simulink model "Kinarm_Approach_Avoidance_Task"  (R2019b)
settings: Solver=ode4  StartTime=0.0  StopTime=inf  FixedStep=BKIN_STEP_TIME  RelTol=1e-3  EnableMultiTasking=on
StartFcn:
  |  warndlg('Dexterit-E models cannot run under simulation. Please compile your model and run it from within Dexterit-E.');set_param(bdroot,'SimulationCommand','stop')
model workspace (MAT data in the model file):
  ADJUST_START = 2
  APPROACH_TARGET_COL = 6
  AVOID_DIST_ADJUST = 6
  AVOID_TARGET_COL = 2
  BEGIN_TARGET_COL = 3
  BKIN_KINEMATIC_FRAME_SIZE = 400
  BKIN_STEP_TIME = 0.00025
  COLOUR_2ND = 7
  COLOUR_3RD = 11
  COLOUR_4TH = 12
  COLOUR_INIT = 6
  CS_OR_AS = 7
  ERROR_DELAY = 10
  E_ACTIVE_APP = 24
  E_APPROACHED = 19
  E_AVOIDED = 21
  E_CIRCLE_APP = 26
  E_ERROR_TRIAL = 23
  E_HAND_IN_START = 17
  E_HAND_LEFT = 16
  E_LEFT_TARG_ON = 2
  E_LOC_1 = 3
  E_LOC_10 = 12
  E_LOC_11 = 13
  E_LOC_12 = 14
  E_LOC_2 = 4
  E_LOC_3 = 5
  E_LOC_4 = 6
  E_LOC_5 = 7
  E_LOC_6 = 8
  E_LOC_7 = 9
  E_LOC_8 = 10
  E_LOC_9 = 11
  E_NO_EVENT = 0
  E_RIGHT_TARG_ON = 1
  E_SEDEN_APP = 25
  E_SQUARE_APP = 27
  E_TARGET_ON = 18
  E_TIMED_OUT = 22
  E_TRIAL_END = 20
  E_TRIAL_START = 15
  INFO_TARGET_COL = 5
  LABEL_COL = 4
  LABEL_HEIGHT = 9
  LABEL_TEXT = 8
  LENGTH = 3
  MAX_FORCE = 3
  MAX_FORCE_BG = 4
  RADIUS_VIS = 3
  RAMP_DURATION = 5
  RAND_START_DELAY = 8
  REACH_TIME = 11
  START_HOLD_DELAY = 7
  START_TARGET_COL = 1
  STROKE_WIDTH = 10
  SUCCESS_DELAY = 9
  TARGET_X = 4
  TARGET_Y = 5
  TARG_DIST = 1
  TARG_LENGTH = 3
  TARG_WIDTH = 4
  TOGGLE_FIELD = 8
  TRIAL_TIME = 12
  WIDTH = 4
  Width = 4
  col_x = 1
  col_y = 2
undefined symbols (not defined in the file): slselsubs
libraries: Video x7, General x3, KINARM_general x3, KINARM_EP_loads x3
settings Model: ModifiedComment=chris -- Wed Feb 16 09:18:30 2005 -- Version 1.1384  ModifiedHistory=Feb 16/05 - Add error repeat, add offset ramp  ExtModeArmWhenConnect=off  ExtModeLogAll=off  OrderedModelArguments=off  Creator=Chris Grebeldinger  LastModifiedBy=User
settings SolverCC: AutoInsertRateTranBlk=on
settings DataIOCC: SaveFormat=Array  SignalLoggingSaveFormat=ModelDataLogs  SaveOutput=off  SaveTime=off  ReturnWorkspaceOutputs=off  SignalLoggingName=sigsOut
settings OptimizationCC: BlockReduction=off  BooleanDataType=off  OptimizeBlockIOStorage=off  BufferReuse=off  GlobalBufferReuse=off  ExpressionFolding=off  ExpressionDepthLimit=2147483647  LocalBlockOutputs=off  InitFltsAndDblsToZero=on  LifeSpan=inf  OptimizeDataStoreBuffers=off  BusAssignmentInplaceUpdate=off
settings DebuggingCC: SaveWithParameterizedLinksMsg=none  UnderspecifiedInitializationDetection=Classic  MergeDetectMultiDrivingBlocksExec=none  SignalResolutionControl=TryResolveAllWithWarning  MultiTaskDSMMsg=warning  FcnCallInpInsideContextMsg=warning  BusObjectLabelMismatch=none  StateNameClashWarn=warning  StrictBusMsg=ErrorOnBusTreatedAsVector  SFUnexpectedBacktrackingDiag=warning  SFNoUnconditionalDefaultTransitionDiag=warning  SFExecutionAtInitializationDiag=none  ArithmeticOperatorsInVariantConditions=warning
settings HardwareCC: ProdBitPerPointer=32  ProdBitPerSizeT=32  ProdBitPerPtrDiffT=32  ProdLargestAtomicFloat=None  ProdWordSize=32  ProdLongLongMode=on  ProdHWDeviceType=Generic->32-bit x86 compatible  TargetLongLongMode=on  TargetIntDivRoundTo=Zero  TargetEndianess=LittleEndian  TargetHWDeviceType=Generic->32-bit x86 compatible
settings ModelReferenceCC: PropagateSignalLabelsOutOfModel=off
settings SFSimCC: SimCustomHeaderCode="#include \"stdlib.h\""  SimUseLocalCustomCode=off  SimParseCustomCode=off  CustomCodeUndefinedFunction=UseInterfaceOnly
settings RTWCC: Description=Simulink Real-Time  SystemTargetFile=slrt.tlc  TemplateMakefile=slrt_default_tmf  RTWUseLocalCustomCode=off  CustomSourceCode="#include \"stdlib.h\""  CodeExecutionProfiling=on
settings CodeAppCC: MaxIdLength=63  StateflowObjectComments=on
settings SimulinkRealTimeCC: TargetFcnLib=ansi_tfl_tmw.mat  GeneratePreprocessorConditionals=Disable all  PreserveStateflowLocalDataDimensions=off
settings ConfigComp: CovMetricSettings=dw  CovHtmlReporting=on  CovSaveCumulativeToWorkspaceVar=on  CovSaveSingleToWorkspaceVar=on  CovExternalEMLEnable=off

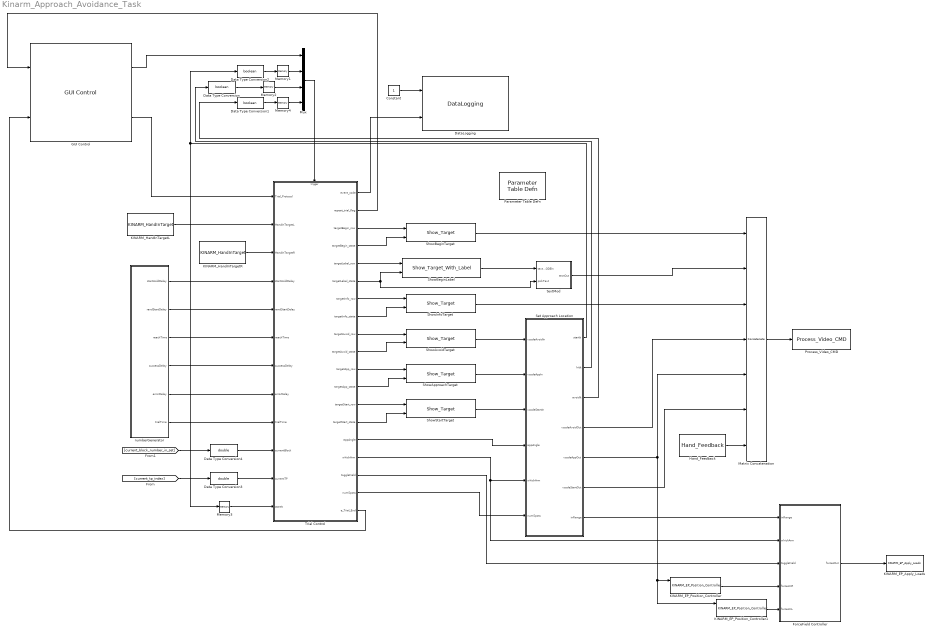
== system Kinarm_Approach_Avoidance_Task ==
  Constant : Constant
  Data Type Conversion : DataTypeConversion  OutDataTypeStr=boolean
  Data Type Conversion1 : DataTypeConversion  OutDataTypeStr=boolean
  Data Type Conversion2 : DataTypeConversion  OutDataTypeStr=boolean
  Data Type Conversion3 : DataTypeConversion  OutDataTypeStr=double
  Data Type Conversion4 : DataTypeConversion  OutDataTypeStr=double
  DataLogging : General/DataLogging  log_event_codes=on  log_analog_inputs=off  show_time_remaining=off  ecat_include=on
  ForceField Controller : Subsystem
  GUI Control : General/GUI Control  task_version=1.0  show_repeat_trial_flag=on  use_custom_tp=off  target_type_str=Circle  Target_Type=1  XYcols=[1 2]  Vcols=3  Lcols=4  indices_padding=[0 0 0 0;0 0 0 0]  target_table_rows=64  load_table_rows=20  tp_table_rows=100
  Hand_Feedback : KINARM_general/Hand_Feedback  feedback_cntl_src=none
  KINARM_EP_Apply_Loads : KINARM_EP_loads/KINARM_EP_Apply_Loads  up_duration=1500  down_duration=1500  max_force=30
  KINARM_EP_Position_Controller : KINARM_EP_loads/KINARM_EP_Position_Controller  use_dom_hand=on  inertias_for_FF=KINARM End Point robot  gain_choice=Standard Movement  sample_time=0.001
  KINARM_EP_Position_Controller1 : KINARM_EP_loads/KINARM_EP_Position_Controller  use_dom_hand=off  inertias_for_FF=KINARM End Point robot  gain_choice=Standard Movement  sample_time=0.001
  KINARM_HandInTargetL : KINARM_general/KINARM_HandInTarget  use_dominant_hand=off  target_type=Circle  num_states=1  attribcol1=[RADIUS_VIS]  attribcol2=[0]  attribcol3=[0]  attribcol4=[0]  attribcol5=[0]
  KINARM_HandInTargetR : KINARM_general/KINARM_HandInTarget  use_dominant_hand=on  target_type=Circle  num_states=1  attribcol1=[RADIUS_VIS]  attribcol2=[0]  attribcol3=[0]  attribcol4=[0]  attribcol5=[0]
  Matrix Concatenation : Concatenate  NumInputs=7  Mode=Multidimensional array
  Memory{1..4} (4 alike) : Memory
  Mux : Mux
  Parameter Table Defn : General/Parameter Table Defn  ShowInLibBrowser=0
  Process_Video_CMD : Video/Process_Video_CMD  video_delay=50
  Set Approach Location : Subsystem
  ShowApproachTarget : Video/Show_Target  target_type=Circle  num_states=1  attribcol1=[COLOUR_INIT 0 0 RADIUS_VIS]  attribcol2=[0 0 0 0]  attribcol3=[0 0 0 0]  attribcol4=[0 0 0 0]  attribcol5=[0 0 0 0]  stateindices_padding=[0 0 0 0 0 0 0;0 0 0 0 0 0 0;0 0 0 0 0 0 0;0 0 0 0 0 0 0;0 0 0 0 0 0 0]  source=dialog  opacity=100  target_display=Both subject and operator displays  num_col=4
  ShowAvoidTarget : Video/Show_Target  target_type=Circle  num_states=1  attribcol1=[COLOUR_INIT COLOUR_2ND STROKE_WIDTH RADIUS_VIS]  attribcol2=[0 0 0 0]  attribcol3=[0 0 0 0]  attribcol4=[0 0 0 0]  attribcol5=[0 0 0 0]  stateindices_padding=[0 0 0 0 0 0 0;0 0 0 0 0 0 0;0 0 0 0 0 0 0;0 0 0 0 0 0 0;0 0 0 0 0 0 0]  source=dialog  opacity=100  target_display=Both subject and operator displays  num_col=4
  ShowBeginLabel : Video/Show_Target_With_Label  target_type=Circle  num_states=3  attribcol1=[0 0 0 0 LABEL_TEXT COLOUR_INIT LABEL_HEIGHT]  attribcol2=[0 0 0 0 LABEL_TEXT COLOUR_2ND LABEL_HEIGHT]  attribcol3=[0 0 0 0 LABEL_TEXT COLOUR_3RD LABEL_HEIGHT]  attribcol4=[0 0 0 0 0 0 0]  attribcol5=[0 0 0 0 0 0 0]  stateindices_padding=[0 0 0 0;0 0 0 0;0 0 0 0;0 0 0 0;0 0 0 0]  source=dialog  opacity=100  target_display=Both subject and operator displays
  ShowBeginTarget : Video/Show_Target  target_type=Circle  num_states=1  attribcol1=[COLOUR_INIT COLOUR_2ND STROKE_WIDTH RADIUS_VIS]  attribcol2=[0 0 0 0]  attribcol3=[0 0 0 0]  attribcol4=[0 0 0 0]  attribcol5=[0 0 0 0]  stateindices_padding=[0 0 0 0 0 0 0;0 0 0 0 0 0 0;0 0 0 0 0 0 0;0 0 0 0 0 0 0;0 0 0 0 0 0 0]  source=dialog  opacity=100  target_display=Both subject and operator displays  num_col=4
  ShowInfoTarget : Video/Show_Target  target_type=Rectangle  num_states=4  attribcol1=[COLOUR_INIT 0 0 TARGET_X TARGET_Y 0]  attribcol2=[COLOUR_2ND 0 0 TARGET_X TARGET_Y 0]  attribcol3=[COLOUR_3RD 0 0 TARGET_X TARGET_Y 0]  attribcol4=[COLOUR_4TH 0 0 TARGET_X TARGET_Y 0]  attribcol5=[0 0 0 0 0 0]  stateindices_padding=[0 0 0 0 0;0 0 0 0 0;0 0 0 0 0;0 0 0 0 0;0 0 0 0 0]  source=dialog  opacity=100  target_display=Both subject and operator displays  num_col=6
  ShowStartTarget : Video/Show_Target  target_type=Circle  num_states=1  attribcol1=[COLOUR_INIT 0 0 RADIUS_VIS]  attribcol2=[0 0 0 0]  attribcol3=[0 0 0 0]  attribcol4=[0 0 0 0]  attribcol5=[0 0 0 0]  stateindices_padding=[0 0 0 0 0 0 0;0 0 0 0 0 0 0;0 0 0 0 0 0 0;0 0 0 0 0 0 0;0 0 0 0 0 0 0]  source=dialog  opacity=100  target_display=Both subject and operator displays  num_col=4
  Trial Control : Stateflow chart  TreatAsAtomicUnit=on
  numberGenerator : Subsystem
  textMod : Subsystem
  wires:
  Trial Control/19(e_Trial_End) -> GUI Control/2
  Trial Control/14(targetStart_state) -> ShowStartTarget/2
  Trial Control/13(targetStart_row) -> ShowStartTarget/1
  Matrix Concatenation/1 -> Process_Video_CMD/1
  Trial Control/1(event_code) -> DataLogging/2
  ShowStartTarget/1 -> Set Approach Location/3(vcodeStartIn)
  Constant/1 -> DataLogging/1
  GUI Control/2 -> Trial Control/1(Trial_Protocol)
  Trial Control/11(targetApp_row) -> ShowApproachTarget/1
  Trial Control/12(targetApp_state) -> ShowApproachTarget/2
  Trial Control/2(repeat_trial_flag) -> GUI Control/1
  KINARM_EP_Position_Controller/1 -> ForceField Controller/4(forcesInR)
  GUI Control/1 -> Mux/1
  [current_tp_index] -> Data Type Conversion3/1
  ShowApproachTarget/1 -> Set Approach Location/2(vcodeAppIn)
  Set Approach Location/6(vcodeStartOut) -> Matrix Concatenation/6
  Set Approach Location/5(vcodeAppOut) -> KINARM_EP_Position_Controller/1, KINARM_EP_Position_Controller1/1, Matrix Concatenation/5
  Set Approach Location/4(vcodeAvoidOut) -> Matrix Concatenation/4
  Set Approach Location/1(startIt) -> Memory3/1, Data Type Conversion2/1
  KINARM_EP_Position_Controller1/1 -> ForceField Controller/5(forcesInL)
  Trial Control/15(appAngle) -> Set Approach Location/4(appAngle)
  Trial Control/16(whichArm) -> ForceField Controller/2(whichArm), Set Approach Location/5(whichArm)
  ShowInfoTarget/1 -> Matrix Concatenation/3
  KINARM_HandInTargetR/1 -> Trial Control/3(HandInTargetR)
  KINARM_HandInTargetL/1 -> Trial Control/2(HandInTargetL)
  Trial Control/17(toggleField) -> ForceField Controller/3(toggleField)
  ForceField Controller/1(forcesOut) -> KINARM_EP_Apply_Loads/1
  Trial Control/3(targetBegin_row) -> ShowBeginTarget/1
  Trial Control/4(targetBegin_state) -> ShowBeginTarget/2
  Trial Control/7(targetInfo_row) -> ShowInfoTarget/1
  Trial Control/8(targetInfo_state) -> ShowInfoTarget/2
  Trial Control/5(targetLabel_row) -> ShowBeginLabel/1
  Trial Control/6(targetLabel_state) -> ShowBeginLabel/2, textMod/2(pickText)
  numberGenerator/1(startHoldDelay) -> Trial Control/4(startHoldDelay)
  numberGenerator/2(randStartDelay) -> Trial Control/5(randStartDelay)
  numberGenerator/6(trialTime) -> Trial Control/9(trialTime)
  numberGenerator/3(reachTime) -> Trial Control/6(reachTime)
  numberGenerator/4(successDelay) -> Trial Control/7(successDelay)
  numberGenerator/5(errorDelay) -> Trial Control/8(errorDelay)
  ShowBeginLabel/1 -> textMod/1(textVCODEIn)
  ShowBeginTarget/1 -> Matrix Concatenation/1
  Hand_Feedback/1 -> Matrix Concatenation/7
  Set Approach Location/7(inRange) -> ForceField Controller/1(inRange)
  Mux/1 -> Trial Control/Trigger
  Memory2/1 -> Mux/3
  Memory4/1 -> Mux/4
  Set Approach Location/2(hitIt) -> Data Type Conversion/1
  Set Approach Location/3(avoidIt) -> Data Type Conversion1/1
  Data Type Conversion/1 -> Memory2/1
  Data Type Conversion1/1 -> Memory4/1
  Data Type Conversion2/1 -> Memory1/1
  Memory1/1 -> Mux/2
  Data Type Conversion3/1 -> Trial Control/11(currentTP)
  Trial Control/9(targetAvoid_row) -> ShowAvoidTarget/1
  Trial Control/10(targetAvoid_state) -> ShowAvoidTarget/2
  ShowAvoidTarget/1 -> Set Approach Location/1(vcodeAvoidIn)
  [current_block_number_in_set] -> Data Type Conversion4/1
  Data Type Conversion4/1 -> Trial Control/10(currentBlock)
  Memory3/1 -> Trial Control/12(startIt)
  textMod/1(textOut) -> Matrix Concatenation/2
  Trial Control/18(numSpots) -> Set Approach Location/6(numSpots)

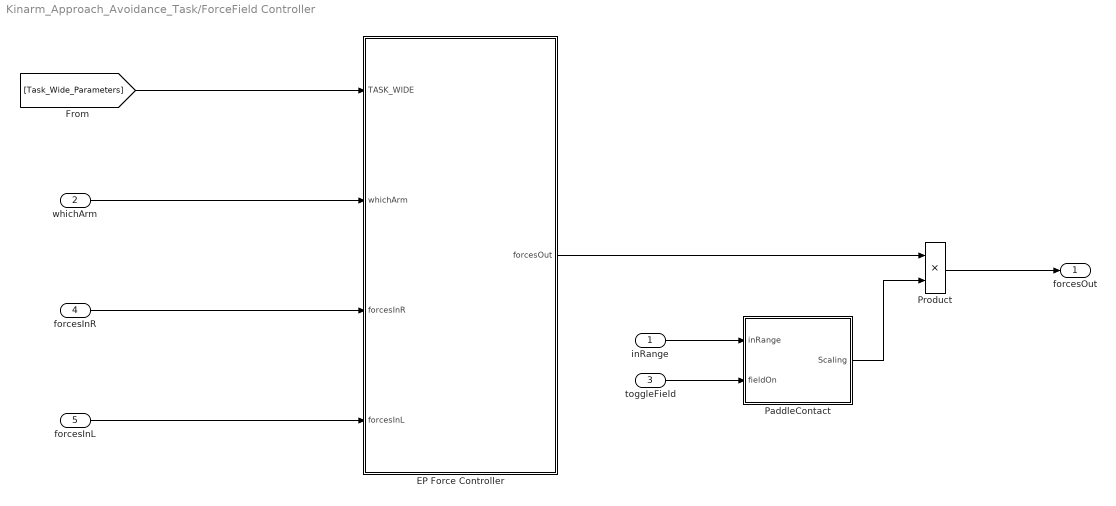
== system Kinarm_Approach_Avoidance_Task/ForceField Controller ==
  inRange : Inport
  whichArm : Inport  Port=2
  toggleField : Inport  Port=3
  forcesInR : Inport  Port=4
  forcesInL : Inport  Port=5
  EP Force Controller : MATLAB Function  TreatAsAtomicUnit=on
  PaddleContact : Subsystem  mask(Perturbation){}
  Product : Product
  forcesOut : Outport
  wires:
  [Task_Wide_Parameters] -> EP Force Controller/1(TASK_WIDE)
  EP Force Controller/1(forcesOut) -> Product/1
  toggleField/1 -> PaddleContact/2(fieldOn)
  forcesInR/1 -> EP Force Controller/3(forcesInR)
  whichArm/1 -> EP Force Controller/2(whichArm)
  forcesInL/1 -> EP Force Controller/4(forcesInL)
  PaddleContact/1(Scaling) -> Product/2
  inRange/1 -> PaddleContact/1(inRange)
  Product/1 -> forcesOut/1

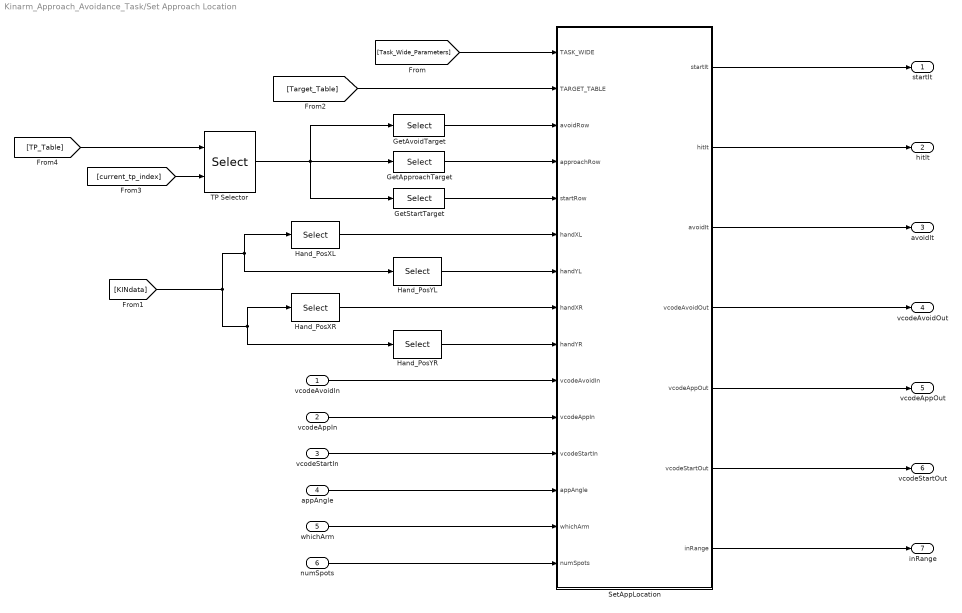
== system Kinarm_Approach_Avoidance_Task/Set Approach Location ==
  vcodeAvoidIn : Inport
  vcodeAppIn : Inport  Port=2
  vcodeStartIn : Inport  Port=3
  appAngle : Inport  Port=4
  whichArm : Inport  Port=5
  numSpots : Inport  Port=6
  GetApproachTarget : Selector  NumberOfDimensions=2  InputPortWidth=3  IndexOptions=Select all,Index vector (dialog)  Indices=[1],[APPROACH_TARGET_COL]  OutputSizes=slselsubs([(-2),(-2)],1),slselsubs([(-2),(-2)],2)
  GetAvoidTarget : Selector  NumberOfDimensions=2  InputPortWidth=3  IndexOptions=Select all,Index vector (dialog)  Indices=[1],[AVOID_TARGET_COL]  OutputSizes=slselsubs([(-2),(-2)],1),slselsubs([(-2),(-2)],2)
  GetStartTarget : Selector  NumberOfDimensions=2  InputPortWidth=3  IndexOptions=Select all,Index vector (dialog)  Indices=[1],[START_TARGET_COL]  OutputSizes=slselsubs([(-2),(-2)],1),slselsubs([(-2),(-2)],2)
  Hand_PosXL : Selector  NumberOfDimensions=2  InputPortWidth=3  IndexOptions=Index vector (dialog),Index vector (dialog)  Indices=[2],[23]  OutputSizes=slselsubs([(-2),(-2)],1),slselsubs([(-2),(-2)],2)
  Hand_PosXR : Selector  NumberOfDimensions=2  InputPortWidth=3  IndexOptions=Index vector (dialog),Index vector (dialog)  Indices=[1],[23]  OutputSizes=slselsubs([(-2),(-2)],1),slselsubs([(-2),(-2)],2)
  Hand_PosYL : Selector  NumberOfDimensions=2  InputPortWidth=3  IndexOptions=Index vector (dialog),Index vector (dialog)  Indices=[2],[24]  OutputSizes=slselsubs([(-2),(-2)],1),slselsubs([(-2),(-2)],2)
  Hand_PosYR : Selector  NumberOfDimensions=2  InputPortWidth=3  IndexOptions=Index vector (dialog),Index vector (dialog)  Indices=[1],[24]  OutputSizes=slselsubs([(-2),(-2)],1),slselsubs([(-2),(-2)],2)
  SetAppLocation : MATLAB Function  TreatAsAtomicUnit=on
  TP Selector : Selector  NumberOfDimensions=2  InputPortWidth=3  IndexOptions=Index vector (port),Select all  Indices=1,-1  OutputSizes=slselsubs([(-2),(-2)],1),slselsubs([(-2),(-2)],2)
  startIt : Outport
  hitIt : Outport  Port=2
  avoidIt : Outport  Port=3
  vcodeAvoidOut : Outport  Port=4
  vcodeAppOut : Outport  Port=5
  vcodeStartOut : Outport  Port=6
  inRange : Outport  Port=7
  wires:
  [Task_Wide_Parameters] -> SetAppLocation/1(TASK_WIDE)
  [current_tp_index] -> TP Selector/2
  Hand_PosXL/1 -> SetAppLocation/6(handXL)
  Hand_PosYL/1 -> SetAppLocation/7(handYL)
  [TP_Table] -> TP Selector/1
  TP Selector/1 -> GetStartTarget/1, GetApproachTarget/1, GetAvoidTarget/1
  GetApproachTarget/1 -> SetAppLocation/4(approachRow)
  [Target_Table] -> SetAppLocation/2(TARGET_TABLE)
  SetAppLocation/2(hitIt) -> hitIt/1
  vcodeAvoidIn/1 -> SetAppLocation/10(vcodeAvoidIn)
  SetAppLocation/4(vcodeAvoidOut) -> vcodeAvoidOut/1
  vcodeAppIn/1 -> SetAppLocation/11(vcodeAppIn)
  vcodeStartIn/1 -> SetAppLocation/12(vcodeStartIn)
  SetAppLocation/5(vcodeAppOut) -> vcodeAppOut/1
  SetAppLocation/6(vcodeStartOut) -> vcodeStartOut/1
  GetAvoidTarget/1 -> SetAppLocation/3(avoidRow)
  GetStartTarget/1 -> SetAppLocation/5(startRow)
  Hand_PosXR/1 -> SetAppLocation/8(handXR)
  Hand_PosYR/1 -> SetAppLocation/9(handYR)
  [KINdata] -> Hand_PosYL/1, Hand_PosXL/1, Hand_PosYR/1, Hand_PosXR/1
  SetAppLocation/1(startIt) -> startIt/1
  SetAppLocation/3(avoidIt) -> avoidIt/1
  whichArm/1 -> SetAppLocation/14(whichArm)
  appAngle/1 -> SetAppLocation/13(appAngle)
  numSpots/1 -> SetAppLocation/15(numSpots)
  SetAppLocation/7(inRange) -> inRange/1

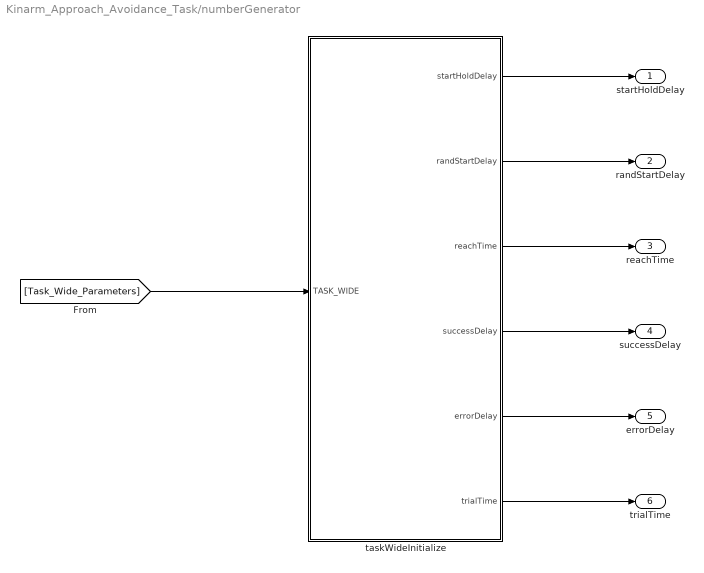
== system Kinarm_Approach_Avoidance_Task/numberGenerator ==
  taskWideInitialize : MATLAB Function  TreatAsAtomicUnit=on
  startHoldDelay : Outport
  randStartDelay : Outport  Port=2
  reachTime : Outport  Port=3
  successDelay : Outport  Port=4
  errorDelay : Outport  Port=5
  trialTime : Outport  Port=6
  wires:
  [Task_Wide_Parameters] -> taskWideInitialize/1(TASK_WIDE)
  taskWideInitialize/1(startHoldDelay) -> startHoldDelay/1
  taskWideInitialize/2(randStartDelay) -> randStartDelay/1
  taskWideInitialize/6(trialTime) -> trialTime/1
  taskWideInitialize/3(reachTime) -> reachTime/1
  taskWideInitialize/4(successDelay) -> successDelay/1
  taskWideInitialize/5(errorDelay) -> errorDelay/1

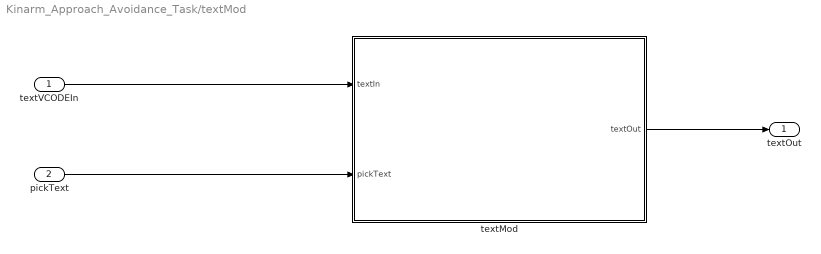
== system Kinarm_Approach_Avoidance_Task/textMod ==
  textVCODEIn : Inport
  pickText : Inport  Port=2
  textMod : MATLAB Function  TreatAsAtomicUnit=on
  textOut : Outport
  wires:
  textMod/1(textOut) -> textOut/1
  textVCODEIn/1 -> textMod/1(textIn)
  pickText/1 -> textMod/2(pickText)

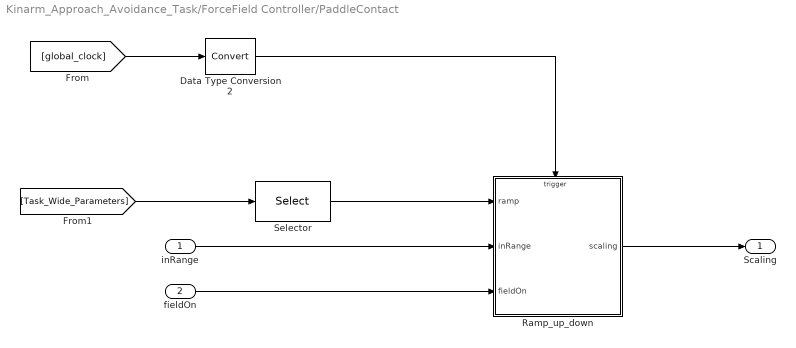
== system Kinarm_Approach_Avoidance_Task/ForceField Controller/PaddleContact ==
  inRange : Inport
  fieldOn : Inport  Port=2
  Data Type Conversion2 : DataTypeConversion
  Ramp_up_down : Stateflow chart  TreatAsAtomicUnit=on
  Selector : Selector  NumberOfDimensions=2  InputPortWidth=3  IndexOptions=Index vector (dialog),Select all  Indices=[RAMP_DURATION],[3]  OutputSizes=slselsubs([(-2),(-2)],1),1
  Scaling : Outport
  wires:
  Ramp_up_down/1(scaling) -> Scaling/1
  [global_clock] -> Data Type Conversion2/1
  Data Type Conversion2/1 -> Ramp_up_down/Trigger
  [Task_Wide_Parameters] -> Selector/1
  Selector/1 -> Ramp_up_down/1(ramp)
  inRange/1 -> Ramp_up_down/2(inRange)
  fieldOn/1 -> Ramp_up_down/3(fieldOn)

== matlab function Kinarm_Approach_Avoidance_Task/Set Approach Location/SetAppLocation ==
  data: startIt output; hitIt output; avoidIt output; vcodeAvoidOut output; vcodeAppOut output; vcodeStartOut output; TASK_WIDE input; TARGET_TABLE input; avoidRow input; approachRow input; startRow input; handXL input; handYL input; handXR input; handYR input; vcodeAvoidIn input; vcodeAppIn input; vcodeStartIn input; appAngle input; whichArm input; numSpots input; TARG_DIST parameter; RADIUS_VIS parameter; ADJUST_START parameter; inRange output
function [startIt, hitIt, avoidIt, vcodeAvoidOut, vcodeAppOut, vcodeStartOut, inRange] = fcn...
    (TASK_WIDE, TARGET_TABLE, avoidRow, approachRow, startRow, handXL, handYL, handXR, handYR, vcodeAvoidIn, vcodeAppIn, vcodeStartIn, appAngle, whichArm, numSpots,...
    TARG_DIST, RADIUS_VIS, ADJUST_START)
%This function checks if the hand is in start, approach, or avoid targets.

%% initialize hand and location to be displayed
targDist = TASK_WIDE(TARG_DIST); %gets distance of targets set from task wide
adjustStart = TASK_WIDE(ADJUST_START); %adjusts the left and right distance from the midline for the center of start/approach/avoid targets
angleArray = [0:2*pi/numSpots:2*pi-2*pi/numSpots]; %get radians for each location

%assume hand is right hand being tested
handX = handXR;
handY = handYR;
whichLoc = angleArray(appAngle); %get the location

if (whichArm == 1) %1 is left arm, left arm is being tested
	adjustStart = -TASK_WIDE(ADJUST_START); %shift target center to the left
    handX = handXL;
    handY = handYL;
end

%% initialize radius

rValStart = TARGET_TABLE(startRow,RADIUS_VIS)*0.01; %radius of start target
rValApp = TARGET_TABLE(approachRow,RADIUS_VIS)*0.01; %radius of approach target
rValApp2 = targDist*0.01-rValStart; %radius of force field around approach target accounts for starting target
rValAvoid = TARGET_TABLE(avoidRow,RADIUS_VIS)*0.01; %radius of avoid target

%% change vcodes for start target contact
%Checks if hand is inside of start target (circle) and shamelessly stolen 
%from HandInTarget block and simplified.
vcodeStartOut = vcodeStartIn;

vcodeStartOut(3) = vcodeStartIn(3) + adjustStart*0.01; %x position adjusted depending on arm assessed
vcodeStartOut(4) = vcodeStartIn(4);

deltaxStart=handX-vcodeStartOut(3); %find difference between hand and approach target
deltayStart=handY-vcodeStartOut(4);

distanceStart = deltaxStart.^2 + deltayStart.^2;

if (distanceStart <= rValStart^2) %if hand is in start target then trigger start
    startIt = 1;
else
    startIt = 0;
end


%% change vcodes for approach target contact
%Same as above but for approach target (circle).
vcodeAppOut = vcodeAppIn;

vcodeAppOut(3) = vcodeAppIn(3) + targDist*cos(whichLoc)*0.01 + adjustStart*0.01;
vcodeAppOut(4) = vcodeAppIn(4) + targDist*sin(whichLoc)*0.01;

deltaxApp=handX-vcodeAppOut(3);
deltayApp=handY-vcodeAppOut(4);

distanceApp = deltaxApp.^2 + deltayApp.^2;
if (distanceApp < rValApp^2) %if hand inside approach target
    hitIt = 1;
else
    hitIt = 0;
end

if (distanceApp < rValApp2^2) %if hand inside approach target force field
    inRange = 1;
else
    inRange = 0;
end

%% change vcodes for avoid target no contact
%similar to above but checks if hand is inside avoid target (circle)

vcodeAvoidOut = vcodeAvoidIn;

vcodeAvoidOut(3) = vcodeAvoidIn(3) + targDist*cos(whichLoc+pi)*0.01 + adjustStart*0.01;
vcodeAvoidOut(4) = vcodeAvoidIn(4) + targDist*sin(whichLoc+pi)*0.01;

deltaxAvoid=handX-vcodeAvoidOut(3);
deltayAvoid=handY-vcodeAvoidOut(4);

distanceAvoid = deltaxAvoid.^2 + deltayAvoid.^2;
if (distanceAvoid < rValAvoid^2) %if hand inside approach target
    avoidIt = 1;
else
    avoidIt = 0;
end

== stateflow chart Kinarm_Approach_Avoidance_Task/Trial Control ==
  state Initialize/
    %Task checks if the participant reached for a certain trial or avoided
    %a certain trial successfully,
    %blocks must be 48 trials long
    %each block must have the same type of TP (1-12 or 13-24)
    entry:
    targetStart_row = Trial_Protocol(START_TARGET_COL);
    targetStart_state = 0; %target for beginning a trial
    targetApp_state = 0; %approach target
    targetAvoid_state = 0; %avoid target
    targetInfo_row = Trial_Protocol(INFO_TARGET_COL); %image of approach/avoid association
    targetBegin_row = Trial_Protocol(BEGIN_TARGET_COL); %target for beginning a block
    targetLabel_row = Trial_Protocol(LABEL_COL); %target for displaying text
    targetInfo_state = 0;
  state MainTrial
    state outputBlockOrder/
      %pick 0 or 1 based on the TP to approach or avoid CS or AS images
      entry:
      appAvoidCS = mod(currentTP,2);
      appAvoidAS = mod(currentTP,2);
      csCount = 0;
      asCount = 0;
    state StartofTrial/
      %start trial
      entry:
      targetApp_row = Trial_Protocol(APPROACH_TARGET_COL);
      targetAvoid_row = Trial_Protocol(AVOID_TARGET_COL);
      holdStartTime = startHoldDelay + rand()*randStartDelay; %starting delay
      targetStart_state = 1;
      targetApp_state = 0;
      targetAvoid_state = 0;
      toggleField = 0;
      repeat_trial_flag = 0;
      targetBegin_state = 0;
      targetLabel_state = 0;
      targetInfo_state = 0;
      tpCount(currentTP) = tpCount(currentTP) + 1; %increment the tpCount
      [appAngle, whichArm, numSpots] = arraySetup(tpCount,currentTP); %call the random array of values
      event_code = 1 + whichArm; %send out event code to identify arm
    state csCount/
      entry:
      %sets the circle square condition
      csCount = csCount + 1;
      appAvoid = appAvoidCS;
      %event codes 26 and 27 output circle square instruction images
      event_code = 26+appAvoid;
      %info states 3 and 4 show circle square instruction images
      targetInfo_state = 3+appAvoid;
    state blockStart/
      %show block start targets and note block
      entry:
      blockCheck = currentBlock;
      targetBegin_state = 1;
      targetLabel_state = 1;
      tpCount = zeros(1,24);
    state left/
      %event code for hand leaving start
      entry:
      event_code = E_HAND_LEFT;
    state asCount/
      entry:
      %sets the active sedentary condition
      asCount = asCount + 1;
      appAvoid = appAvoidAS;
      %eventcode 24 and 25 output active seden instruction images
      event_code = 24+appAvoid;
      %info states 1 and 2 show active avoid instruction images
      targetInfo_state = 1+appAvoid;
    state whichSide/
      entry:
      event_code = E_HAND_IN_START;
    state Approached/
      %hand is in approach
      entry:
      event_code = E_APPROACHED;
      toggleField = 0;
    state AppOn/
      %turn on targets for reaching
      entry:
      event_code = 2 + appAngle; %send out event for location
      toggleField = Trial_Protocol(TOGGLE_FIELD); %check if trial has forcefield
      targetStart_state = 0;
      targetApp_state = 1;
      targetAvoid_state = 1;
    state Avoided/
      %hand left avoid target
      entry:
      event_code = E_AVOIDED;
      toggleField = 0;
    state checkError/
      %send out an error for being bad
      entry:
      event_code = E_ERROR_TRIAL;
      targetLabel_state = 2;
    state TimedOut/
      %too slow to reach start/app/avoid
      entry:
      event_code = E_TIMED_OUT;
      targetLabel_state = 3;
      toggleField = 0;
    state EndOfTrial/
      % Turn off targets,
      entry:
      targetStart_state = 0;
      targetAvoid_state = 0;
      targetApp_state = 0;
      toggleField = 0;
    (junction 357) -> outputBlockOrder [order 2] : %if second CS block finished
        | [csCount == 2]
    (junction 355) -> outputBlockOrder [order 2] : %if second AS block finished
        | [asCount == 2]
    outputBlockOrder -> blockStart
    blockStart -> csCount [order 2] : %if circle or square block
        | [Trial_Protocol(CS_OR_AS) == 0]
    (junction 377) -> StartofTrial [order 2] : %if left hand is in begin target
        | [HandInTargetL(targetBegin_row) == 1]
    csCount -> (junction 377)
    (junction 357) -> blockStart [order 1] : %if no CS block finished
        | [csCount == 0]
    (junction 377) -> StartofTrial [order 1] : %if right hand is in begin target
        | [HandInTargetR(targetBegin_row) == 1]
    StartofTrial -> (junction 394)
    (junction 357) -> blockStart [order 3] : %if first CS block finished
        | [csCount == 1]
        | %swap the approach avoid condition
        | {appAvoidCS = 1-appAvoidCS;}
    (junction 355) -> blockStart [order 1] : %if no AS block finished
        | [asCount == 0]
    (junction 355) -> blockStart [order 3] : %if first AS block finished
        | [asCount == 1]
        | %swap the approach avoid condition
        | {appAvoidAS = 1-appAvoidAS;}
    blockStart -> asCount [order 1] : %if active or sedentary block
        | [Trial_Protocol(CS_OR_AS) == 1]
    asCount -> (junction 377)
    left -> (junction 394)
    (junction 394) -> TimedOut [order 1] : %delay for getting to start
        | after(trialTime, msec)
    (junction 394) -> whichSide [order 2] : %checks if hand is
        | %in start
        | [startIt == 1]
    (junction 323) -> (junction 357) [order 2] : %if circle or square block
        | [Trial_Protocol(CS_OR_AS) == 0]
    whichSide -> left [order 1] : %check if hand
        | %left start
        | [startIt == 0]
    (junction 323) -> (junction 355) [order 1] : %if active or sedentary block
        | [Trial_Protocol(CS_OR_AS) == 1]
    whichSide -> AppOn [order 2] : %hand in start delay
        | after(holdStartTime,msec)
    Approached -> checkError [order 1] : %approach to negative stimulus was incorrect during avoid block
        | [(Trial_Protocol(TOGGLE_FIELD) == 1) && appAvoid == 1]
    AppOn -> Approached [order 1] : %check if hit
        | e_hit
    Approached -> checkError [order 3] : %approach to positive stimulus was incorrect during approach block
        | [(Trial_Protocol(TOGGLE_FIELD) == 0) && appAvoid == 0]
    Approached -> EndOfTrial [order 2] : %delay after successful trial
        | after(successDelay,msec)
    AppOn -> Avoided [order 2] : %check if avoided
        | e_avoid
    AppOn -> TimedOut [order 3] : %delay for reaching to target
        | after(reachTime, msec)
    Avoided -> checkError [order 1] : %avoid to negative stimulus was incorrect during approach block
        | [(Trial_Protocol(TOGGLE_FIELD) == 1) && appAvoid == 0]
    Avoided -> checkError [order 3] : %avoid to positive stimulus was incorrect during avoid block
        | [(Trial_Protocol(TOGGLE_FIELD) == 0) && appAvoid == 1]
    Avoided -> EndOfTrial [order 2] : %delay after successful trial
        | after(successDelay,msec)
    checkError -> EndOfTrial : %delay after error trial
        | after(errorDelay,msec)
    TimedOut -> EndOfTrial : %delay after error trial
        | after(errorDelay,msec)
  state Inter_Trial_State/
    %close all
    entry:
    event_code = 0;
    toggleField = 0;
    targetApp_state = 0;
    targetStart_state = 0;
    targetAvoid_state = 0;
    targetLabel_state = 0;
    repeat_trial_flag = 0;
    e_Trial_End;
  state RepeatTrial/
    entry:
    repeat_trial_flag = 1;
  (default) -> Initialize
  (junction 173) -> StartofTrial [order 1] : %keep the trials flowing if the block hasn't changed
      | [currentBlock == blockCheck]
  Initialize -> outputBlockOrder : %wait for task to start
      | [currentTP > 0]
  (junction 173) -> (junction 323) [order 2] : %check if next block is different from last block
      | [currentBlock ~= blockCheck]
  Inter_Trial_State -> (junction 173) : %arbitrary delay
      | after(successDelay,msec)
  RepeatTrial -> Inter_Trial_State : after(1,msec)
  MainTrial -> RepeatTrial : e_ExitTrialNow/
      | {tickCount = 1;}
      | % e_ExitTrialNow event occurs if the
      | % Dex pause is pressed by the operator
  EndOfTrial -> Inter_Trial_State : after(1, msec)
  data: outLoc function_output; outArm function_output; numberLoc function_output; rangeTP function_input; nowTP function_input; event_code output [0..]; repeat_trial_flag output; targetBegin_row output double; targetBegin_state output; targetLabel_row output; targetLabel_state output; targetInfo_row output; targetInfo_state output; targetAvoid_row output; targetAvoid_state output; targetApp_row output [1..32]; targetApp_state output; targetStart_row output; targetStart_state output; appAngle output; whichArm output; tickCount local; Trial_Protocol input; toggleField output; numSpots output; HandInTargetL input; HandInTargetR input; startHoldDelay input; pointer local; randStartDelay input; tpCount local; reachTime input; successDelay input; errorDelay input; trialTime input; holdStartTime local; currentBlock input; blockCheck local; appAvoidCS local; currentTP input; asCount local; csCount local; appAvoidAS local; appAvoid local; startIt input; rndArm local; rndLoc local; rndPointer local
  data targetApp_row settings: description=index of the row currently being used in the TargetTable
  events: e_clk input RISING_EDGE_EVENT; e_ExitTrialNow input RISING_EDGE_EVENT; e_start input RISING_EDGE_EVENT; e_Trial_End output EITHER_EDGE_EVENT; e_avoid input RISING_EDGE_EVENT; e_hit input RISING_EDGE_EVENT
  function [outLoc, outArm, numberLoc] = arraySetup(rangeTP,nowTP):
    | function [outLoc, outArm, numberLoc] = arraySetup(rangeTP,nowTP)
    | %This function sets up a pseudorandom order for the location of targets and
    | %which arm gets tested (numSpots must be set to 12 and numRows needs to 
    | %account for the number of trials, i think 16 is fine)
    | 
    | %% set up random arrays for location and arm
    | %Random arrays are generated that put each of the approach and avoid
    | %targets in 1 of 12 locations for each arm.
    | %Lots of work was done so that each location and arm has at least 1
    | %approach and 1 avoid trial.
    | 
    | numberLoc = 12; %number of trial protocols run
    | numberArm = 2;
    | numberSpots = numberLoc*numberArm;
    | %there are a total of 24 different spots (12 locations for 2 arms) that 2 
    | %different targets (approach or avoid) can appear necessitating 48 trials
    | %for each block
    | 
    | armLoc = zeros(2,numberSpots);
    | armLoc(1,:) = [1:numberSpots/2,1:numberSpots/2]; %which location (1 is east, 4 is north, 7 is west, 10 is south)
    | armLoc(2,:) = [zeros(1,numberSpots/2),ones(1,numberSpots/2)]; %which arm (0 = right,1 = left)
    | persistent atTime0 randPointer
    | if (isempty(atTime0))
    |     atTime0 = 0;
    |     randPointer = [randperm(numberSpots);
    |                     randperm(numberSpots);
    |                     randperm(numberSpots);
    |                     randperm(numberSpots);];
    | end
    | 
    | outLoc = 0;
    | outArm = 0;
    | 
    | activeImageTP = numberSpots/4;
    | sedenImageTP = numberSpots/2;
    | circImageTP = numberSpots*3/4;
    | squareImageTP = numberSpots;
    | 
    | allActive = sum(rangeTP(1:activeImageTP));
    | allSeden = sum(rangeTP(activeImageTP+1:sedenImageTP));
    | allCirc = sum(rangeTP(sedenImageTP+1:circImageTP));
    | allSqu = sum(rangeTP(circImageTP+1:squareImageTP));
    | 
    | if (nowTP <= activeImageTP) %active image currently set to have 6 trials of each type
    |     outLoc = armLoc(1,randPointer(1,allActive));
    |     outArm = armLoc(2,randPointer(1,allActive));
    | elseif (nowTP > activeImageTP && nowTP <= sedenImageTP) %sedentary image
    |     outLoc = armLoc(1,randPointer(2,allSeden));
    |     outArm = armLoc(2,randPointer(2,allSeden));
    | elseif (nowTP > sedenImageTP && nowTP <= circImageTP)
    |     outLoc = armLoc(1,randPointer(3,allCirc));
    |     outArm = armLoc(2,randPointer(3,allCirc));
    | elseif (nowTP > circImageTP)
    |     outLoc = armLoc(1,randPointer(4,allSqu));
    |     outArm = armLoc(2,randPointer(4,allSqu));
    | end

== matlab function Kinarm_Approach_Avoidance_Task/ForceField Controller/EP Force Controller ==
  data: TASK_WIDE input; whichArm input; MAX_FORCE parameter; forcesInR input; forcesInL input; forcesOut output
function forcesOut  = fcn(TASK_WIDE, whichArm, MAX_FORCE, forcesInR, forcesInL)
%Function applies a load to the arm when the hand leaves the start target
%and the trial is a loaded trial (toggleField == 1).

%% initialize
maxForce = TASK_WIDE(MAX_FORCE);

if (whichArm == 1)
    forcesIn = forcesInL;
else
    forcesIn = forcesInR;
end

%% set forces out
%Send out forces to the appropriate arm also shamelessly stolen.

posCon_force1 = sqrt(forcesIn(1)^2 + forcesIn(2)^2);
posCon_force2 = sqrt(forcesIn(3)^2 + forcesIn(4)^2);

forcesOut = -forcesIn;
% limit the force of arm 1
if posCon_force1 > maxForce
    scaling = maxForce / posCon_force1;
    forcesOut(1:2) = forcesOut(1:2) * scaling;
end

% limit the force of arm 2
if posCon_force2 > maxForce
    scaling = maxForce / posCon_force2;
    forcesOut(3:4) = forcesOut(3:4) * scaling;
end

== matlab function Kinarm_Approach_Avoidance_Task/numberGenerator/taskWideInitialize ==
  data: TASK_WIDE input; startHoldDelay output; randStartDelay output; reachTime output; successDelay output; errorDelay output; trialTime output; START_HOLD_DELAY parameter; RAND_START_DELAY parameter; REACH_TIME parameter; TRIAL_TIME parameter; SUCCESS_DELAY parameter; ERROR_DELAY parameter
function [startHoldDelay, randStartDelay, reachTime, successDelay, errorDelay, trialTime] =...
    fcn(TASK_WIDE, START_HOLD_DELAY, RAND_START_DELAY, REACH_TIME, TRIAL_TIME, SUCCESS_DELAY, ERROR_DELAY)  

%% task wide parameter outputs
startHoldDelay = TASK_WIDE(START_HOLD_DELAY); %base time for holding the start target
randStartDelay = TASK_WIDE(RAND_START_DELAY); %random time added to base time for start target
trialTime = TASK_WIDE(TRIAL_TIME); %time allowed to start trial
successDelay = TASK_WIDE(SUCCESS_DELAY); %time delay after a successful trial
errorDelay = TASK_WIDE(ERROR_DELAY); %time delay after an error trial
reachTime = TASK_WIDE(REACH_TIME); %time allotted to reach for a stimulus

== matlab function Kinarm_Approach_Avoidance_Task/textMod/textMod ==
  data: textIn input; pickText input; textOut output
function textOut  = fcn(textIn, pickText)
%modify the label target to display text

textOut = textIn;
if (pickText == 1) %labeltarget state 1
    str1 = ['Place either hand in the circle to start'];
elseif (pickText == 2) %labeltarget state 2
    str1 = ['Incorrect!'];
elseif (pickText == 3) %labeltarget state 3
    str1 = ['Too slow!'];
else
    str1 = ' ';
end
textOut(1,15:(length(str1)+14))=uint16(str1);  %str in letters

== stateflow chart Kinarm_Approach_Avoidance_Task/ForceField Controller/PaddleContact/Ramp_up_down ==
  state peak/
    entry:
    scaling=1;
  state RampingUp/
    %sigmoidal ramping taken from Ethan Heming and
    %modified by Kayne
    entry:
    tick=0;
    CurrScale=scaling;
    b=ramp/4; % Center at Middle;
    c=ramp/20; % Define Rise Rate;
    during:
    tick++;
    scaling = (1-CurrScale)/(1+exp(-1*(tick-b)/c))+CurrScale;
  state RampingDown/
    entry:
    tick=0;
    CurrScale=scaling;
    b=ramp/4; % Center at Middle;
    c=ramp/20; % Define Drop Rate;
    during:
    tick++;
    scaling = CurrScale*(1-1/(1+exp(-1*(tick-b)/c)));
  state minimum/
    entry:
    scaling=0;
  peak -> RampingDown [order 1] : %check if forcefield is turned off
      | [fieldOn == 0]
  RampingUp -> peak : after(ramp, e_clk)
  peak -> RampingDown [order 2] : %check if hand is outside target
      | [inRange == 0]
  RampingDown -> minimum : after(ramp, e_clk)
  minimum -> RampingUp : %check if hand is in target and
      | %trial has a forcefield
      | [inRange == 1 && fieldOn == 1]
  (default) -> minimum
  data: ramp input double; scaling output double; tick local double; c local double; b local double; CurrScale local double; inRange input double; fieldOn input double
  events: e_clk input RISING_EDGE_EVENT
